simulink model "FOCFullSpeedControl"  (R2020b)
settings: Solver=ode4  StartTime=0.0  StopTime=4  FixedStep=1e-6  RelTol=1e-3
values from neighbouring files (symbols this model uses):
  E = 700    [FOCinit.m]
  f = 0.005    [FOCinit.m]
  J = 0.006    [FOCinit.m]
  Kie = 3 / (t5e * Ke)    (= 216000)    [FOCinit.m]
  Kif = 3 / (t5f * Kf)    (= 254.237288136)    [FOCinit.m]
  Kim = 3 / (t5m * Km)    (= 0.03)    [FOCinit.m]
  Kpe = taue * Kie    (= 2830.4)    [FOCinit.m]
  Kpf = tauf * Kif    (= 14.1242937853)    [FOCinit.m]
  Kpm = taum * Kim    (= 0.036)    [FOCinit.m]
  Lr = 0.075    [FOCinit.m]
  Ls = 0.280    (= 0.28)    [FOCinit.m]
  Msr = 0.118    [FOCinit.m]
  P = 2    [FOCinit.m]
  Rr = 1.35    [FOCinit.m]
  Rs = 7.2    [FOCinit.m]
  Ts = 1/fs    (= 0.0001)    [FOCinit.m]
libraries: mcbcontrolslib x6, slpidlib x4, simulink x1
settings Model: SimulationMode=accelerator  Creator=guillaume  LastModifiedBy=SF54888
settings DataIOCC: ReturnWorkspaceOutputs=off
settings DebuggingCC: ArithmeticOperatorsInVariantConditions=warning
settings SFSimCC: SimUseLocalCustomCode=off  CustomCodeUndefinedFunction=UseInterfaceOnly
settings RTWCC: RTWUseLocalCustomCode=off
settings CodeAppCC: StateflowObjectComments=on

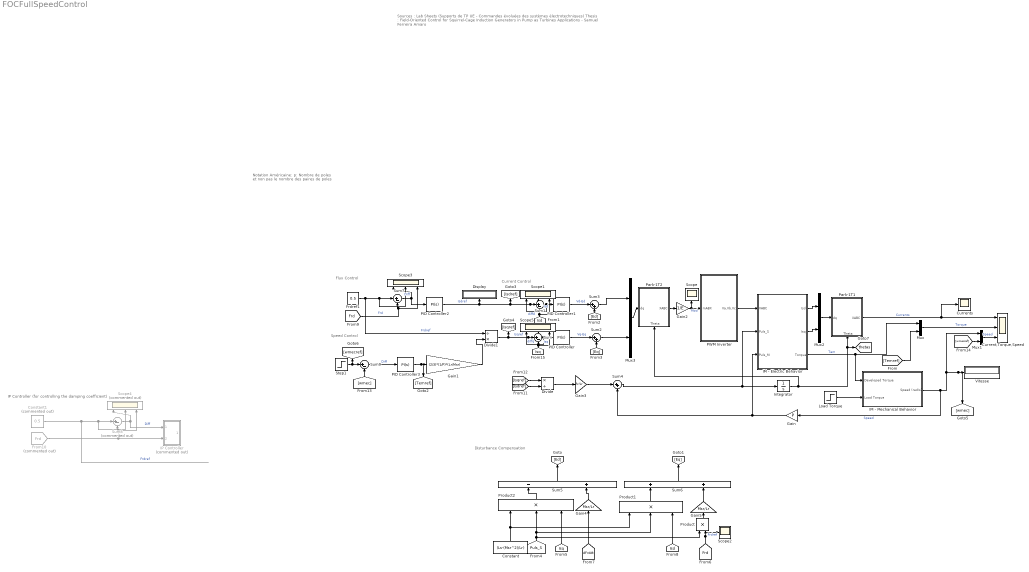
== system FOCFullSpeedControl ==
  note: Sources :
      | Lab Sheets (Supports de TP UE - Commandes évoluées des systèmes électrotechniques)
      | Thesis : Field-Oriented Control for Squirrel-Cage Induction Generators in Pump as Turbines Applications - Samuel Ferreira Amaro
  note: Notation Américaine:
      | p: Nombre de poles et
      | non pas le nombre des paires de poles
  note: Current Control
  note: Disturbance Compensation
  note: Speed Control
  note: IP Controller (for controlling the damping coefficient)
  note: Flux Control
  Constant : Constant  Value=(Ls-(Msr^2)/Lr)
  Constant1 : Constant  Commented=on  Value=0.5
  Current,Torque,Speed : Scope  NumInputPorts=3
  Currents : Scope
  Display : Display
  Divide : Product  Inputs=*/
  Divide1 : Product  Inputs=/*
  Frdref1 : Constant  Value=0.5
  From10 : From  Commented=on  GotoTag=Frd  TagVisibility=global
  Gain : Gain  Gain=P
  Gain1 : Gain  Gain=(2/3)*(1/P)*(Lr/Msr)
  Gain2 : Gain  Gain=1/E
  Gain3 : Gain  Gain=Rr/Lr
  Gain4 : Gain  Gain=Msr/Lr
  Gain5 : Gain  Gain=Msr/Lr
  IM - Electric Behavior : Subsystem
  IM - Mechanical Behavior : Subsystem
  IP Controller : Subsystem  Commented=on
  Integrator : Integrator
  Load Torque : Step  Time=2  After=0.5  SampleTime=0
  Mux{,1..3} (4 alike) : Mux  Inputs=2
  PID Controller : slpidlib/PID Controller  Controller=PI  Form=Parallel  TimeDomain=Continuous-time  UseExternalTs=off  SampleTime=-1  IntegratorMethod=Forward Euler  FilterMethod=Forward Euler  ControllerParametersSource=internal  P=Kpe  I=Kie  D=0  UseFilter=on  N=100  TunerSelectOption=Transfer Function Based (PID Tuner App)  InitialConditionSource=internal  InitialConditionForIntegrator=0  InitialConditionForFilter=0  DifferentiatorICPrevScaledInput=0  ExternalReset=none  TrackingMode=off  Kt=1  LimitOutput=off  SatLimitsSource=internal  UpperSaturationLimit=inf  LowerSaturationLimit=-inf  LinearizeAsGain=on  AntiWindupMode=none  Kb=1  POutMin=[]  POutMax=[]  IOutMin=[]  IOutMax=[]  DOutMin=[]  DOutMax=[]  NOutMin=[]  NOutMax=[]  SumOutMin=[]  SumOutMax=[]  SaturationOutMin=[]  SaturationOutMax=[]  PParamMin=[]  PParamMax=[]  IParamMin=[]  IParamMax=[]  DParamMin=[]  DParamMax=[]  NParamMin=[]  NParamMax=[]  KbParamMin=[]  KbParamMax=[]  KtParamMin=[]  KtParamMax=[]  KbOutMin=[]  KbOutMax=[]  KtOutMin=[]  KtOutMax=[]  IntegratorOutMin=[]  IntegratorOutMax=[]  FilterOutMin=[]  FilterOutMax=[]  SumI1OutMin=[]  SumI1OutMax=[]  SumI2OutMin=[]  SumI2OutMax=[]  SumI3OutMin=[]  SumI3OutMax=[]  SumI4OutMin=[]  SumI4OutMax=[]  SumDOutMin=[]  SumDOutMax=[]  DifferentiatorOutMin=[]  DifferentiatorOutMax=[]  FilterDiffOutCoefMin=[]  FilterDiffOutCoefMax=[]  ReciprocalOutMin=[]  ReciprocalOutMax=[]  SumDenOutMin=[]  SumDenOutMax=[]  SumNumOutMin=[]  SumNumOutMax=[]  DivideOutMin=[]  DivideOutMax=[]  UdiffTsProdOutMin=[]  UdiffTsProdOutMax=[]  NTsProdOutMin=[]  NTsProdOutMax=[]  UintegralTsProdOutMin=[]  UintegralTsProdOutMax=[]  UngainTsProdOutMin=[]  UngainTsProdOutMax=[]  IntegratorContinuousStateAttributes=''  IntegratorStateMustResolveToSignalObject=off  IntegratorRTWStateStorageClass=Auto  FilterContinuousStateAttributes=''  FilterStateMustResolveToSignalObject=off  FilterRTWStateStorageClass=Auto  ParallelPVariant=InternalParameters  IdealPVariant=Disabled  IVariant=InternalParameters  DVariant=Disabled  IntegratorVariant=Continuous  SatVariant=Disabled  AWVariant=Passthrough  PCopyVariant=Disabled  TRVariant=Disabled  FdbkBlocksVariant=Forward  IdealPFdbkVariant=Disabled  SatFdbkVariant=Disabled  DerivativeFilterVariant=Disabled  NVariant=Disabled  NCopyVariant=Disabled_SignalSpec  FilterICVariant=Disabled  IntegratorICVariant=InternalICs  ExternalResetVariant=Disabled  TRSumVariant=Passthrough  SumFdbkVariant=Disabled  SumVariant=Sum_PI  TsampFilterVariant=InternalTs  TsampNgainVariant=Passthrough  TsampIntegralVariant=Passthrough  ExternalSaturationOutDataTypeStr=Inherit: Same as second input
  PID Controller1 : slpidlib/PID Controller  Controller=PI  Form=Parallel  TimeDomain=Continuous-time  UseExternalTs=off  SampleTime=-1  IntegratorMethod=Forward Euler  FilterMethod=Forward Euler  ControllerParametersSource=internal  P=Kpe  I=Kie  D=0  UseFilter=on  N=100  TunerSelectOption=Transfer Function Based (PID Tuner App)  InitialConditionSource=internal  InitialConditionForIntegrator=0  InitialConditionForFilter=0  DifferentiatorICPrevScaledInput=0  ExternalReset=none  TrackingMode=off  Kt=1  LimitOutput=off  SatLimitsSource=internal  UpperSaturationLimit=inf  LowerSaturationLimit=-inf  LinearizeAsGain=on  AntiWindupMode=none  Kb=1  POutMin=[]  POutMax=[]  IOutMin=[]  IOutMax=[]  DOutMin=[]  DOutMax=[]  NOutMin=[]  NOutMax=[]  SumOutMin=[]  SumOutMax=[]  SaturationOutMin=[]  SaturationOutMax=[]  PParamMin=[]  PParamMax=[]  IParamMin=[]  IParamMax=[]  DParamMin=[]  DParamMax=[]  NParamMin=[]  NParamMax=[]  KbParamMin=[]  KbParamMax=[]  KtParamMin=[]  KtParamMax=[]  KbOutMin=[]  KbOutMax=[]  KtOutMin=[]  KtOutMax=[]  IntegratorOutMin=[]  IntegratorOutMax=[]  FilterOutMin=[]  FilterOutMax=[]  SumI1OutMin=[]  SumI1OutMax=[]  SumI2OutMin=[]  SumI2OutMax=[]  SumI3OutMin=[]  SumI3OutMax=[]  SumI4OutMin=[]  SumI4OutMax=[]  SumDOutMin=[]  SumDOutMax=[]  DifferentiatorOutMin=[]  DifferentiatorOutMax=[]  FilterDiffOutCoefMin=[]  FilterDiffOutCoefMax=[]  ReciprocalOutMin=[]  ReciprocalOutMax=[]  SumDenOutMin=[]  SumDenOutMax=[]  SumNumOutMin=[]  SumNumOutMax=[]  DivideOutMin=[]  DivideOutMax=[]  UdiffTsProdOutMin=[]  UdiffTsProdOutMax=[]  NTsProdOutMin=[]  NTsProdOutMax=[]  UintegralTsProdOutMin=[]  UintegralTsProdOutMax=[]  UngainTsProdOutMin=[]  UngainTsProdOutMax=[]  IntegratorContinuousStateAttributes=''  IntegratorStateMustResolveToSignalObject=off  IntegratorRTWStateStorageClass=Auto  FilterContinuousStateAttributes=''  FilterStateMustResolveToSignalObject=off  FilterRTWStateStorageClass=Auto  ParallelPVariant=InternalParameters  IdealPVariant=Disabled  IVariant=InternalParameters  DVariant=Disabled  IntegratorVariant=Continuous  SatVariant=Disabled  AWVariant=Passthrough  PCopyVariant=Disabled  TRVariant=Disabled  FdbkBlocksVariant=Forward  IdealPFdbkVariant=Disabled  SatFdbkVariant=Disabled  DerivativeFilterVariant=Disabled  NVariant=Disabled  NCopyVariant=Disabled_SignalSpec  FilterICVariant=Disabled  IntegratorICVariant=InternalICs  ExternalResetVariant=Disabled  TRSumVariant=Passthrough  SumFdbkVariant=Disabled  SumVariant=Sum_PI  TsampFilterVariant=InternalTs  TsampNgainVariant=Passthrough  TsampIntegralVariant=Passthrough  ExternalSaturationOutDataTypeStr=Inherit: Same as second input
  PID Controller2 : slpidlib/PID Controller  Controller=PI  Form=Parallel  TimeDomain=Continuous-time  UseExternalTs=off  SampleTime=-1  IntegratorMethod=Forward Euler  FilterMethod=Forward Euler  ControllerParametersSource=internal  P=Kpf  I=Kif  D=0  UseFilter=on  N=100  TunerSelectOption=Transfer Function Based (PID Tuner App)  InitialConditionSource=internal  InitialConditionForIntegrator=0  InitialConditionForFilter=0  DifferentiatorICPrevScaledInput=0  ExternalReset=none  TrackingMode=off  Kt=1  LimitOutput=off  SatLimitsSource=internal  UpperSaturationLimit=inf  LowerSaturationLimit=-inf  LinearizeAsGain=on  AntiWindupMode=none  Kb=1  POutMin=[]  POutMax=[]  IOutMin=[]  IOutMax=[]  DOutMin=[]  DOutMax=[]  NOutMin=[]  NOutMax=[]  SumOutMin=[]  SumOutMax=[]  SaturationOutMin=[]  SaturationOutMax=[]  PParamMin=[]  PParamMax=[]  IParamMin=[]  IParamMax=[]  DParamMin=[]  DParamMax=[]  NParamMin=[]  NParamMax=[]  KbParamMin=[]  KbParamMax=[]  KtParamMin=[]  KtParamMax=[]  KbOutMin=[]  KbOutMax=[]  KtOutMin=[]  KtOutMax=[]  IntegratorOutMin=[]  IntegratorOutMax=[]  FilterOutMin=[]  FilterOutMax=[]  SumI1OutMin=[]  SumI1OutMax=[]  SumI2OutMin=[]  SumI2OutMax=[]  SumI3OutMin=[]  SumI3OutMax=[]  SumI4OutMin=[]  SumI4OutMax=[]  SumDOutMin=[]  SumDOutMax=[]  DifferentiatorOutMin=[]  DifferentiatorOutMax=[]  FilterDiffOutCoefMin=[]  FilterDiffOutCoefMax=[]  ReciprocalOutMin=[]  ReciprocalOutMax=[]  SumDenOutMin=[]  SumDenOutMax=[]  SumNumOutMin=[]  SumNumOutMax=[]  DivideOutMin=[]  DivideOutMax=[]  UdiffTsProdOutMin=[]  UdiffTsProdOutMax=[]  NTsProdOutMin=[]  NTsProdOutMax=[]  UintegralTsProdOutMin=[]  UintegralTsProdOutMax=[]  UngainTsProdOutMin=[]  UngainTsProdOutMax=[]  IntegratorContinuousStateAttributes=''  IntegratorStateMustResolveToSignalObject=off  IntegratorRTWStateStorageClass=Auto  FilterContinuousStateAttributes=''  FilterStateMustResolveToSignalObject=off  FilterRTWStateStorageClass=Auto  ParallelPVariant=InternalParameters  IdealPVariant=Disabled  IVariant=InternalParameters  DVariant=Disabled  IntegratorVariant=Continuous  SatVariant=Disabled  AWVariant=Passthrough  PCopyVariant=Disabled  TRVariant=Disabled  FdbkBlocksVariant=Forward  IdealPFdbkVariant=Disabled  SatFdbkVariant=Disabled  DerivativeFilterVariant=Disabled  NVariant=Disabled  NCopyVariant=Disabled_SignalSpec  FilterICVariant=Disabled  IntegratorICVariant=InternalICs  ExternalResetVariant=Disabled  TRSumVariant=Passthrough  SumFdbkVariant=Disabled  SumVariant=Sum_PI  TsampFilterVariant=InternalTs  TsampNgainVariant=Passthrough  TsampIntegralVariant=Passthrough  ExternalSaturationOutDataTypeStr=Inherit: Same as second input
  PID Controller3 : slpidlib/PID Controller  Controller=PI  Form=Parallel  TimeDomain=Continuous-time  UseExternalTs=off  SampleTime=-1  IntegratorMethod=Forward Euler  FilterMethod=Forward Euler  ControllerParametersSource=internal  P=Kpm  I=Kim  D=0  UseFilter=on  N=100  TunerSelectOption=Transfer Function Based (PID Tuner App)  InitialConditionSource=internal  InitialConditionForIntegrator=0  InitialConditionForFilter=0  DifferentiatorICPrevScaledInput=0  ExternalReset=none  TrackingMode=off  Kt=1  LimitOutput=off  SatLimitsSource=internal  UpperSaturationLimit=inf  LowerSaturationLimit=-inf  LinearizeAsGain=on  AntiWindupMode=none  Kb=1  POutMin=[]  POutMax=[]  IOutMin=[]  IOutMax=[]  DOutMin=[]  DOutMax=[]  NOutMin=[]  NOutMax=[]  SumOutMin=[]  SumOutMax=[]  SaturationOutMin=[]  SaturationOutMax=[]  PParamMin=[]  PParamMax=[]  IParamMin=[]  IParamMax=[]  DParamMin=[]  DParamMax=[]  NParamMin=[]  NParamMax=[]  KbParamMin=[]  KbParamMax=[]  KtParamMin=[]  KtParamMax=[]  KbOutMin=[]  KbOutMax=[]  KtOutMin=[]  KtOutMax=[]  IntegratorOutMin=[]  IntegratorOutMax=[]  FilterOutMin=[]  FilterOutMax=[]  SumI1OutMin=[]  SumI1OutMax=[]  SumI2OutMin=[]  SumI2OutMax=[]  SumI3OutMin=[]  SumI3OutMax=[]  SumI4OutMin=[]  SumI4OutMax=[]  SumDOutMin=[]  SumDOutMax=[]  DifferentiatorOutMin=[]  DifferentiatorOutMax=[]  FilterDiffOutCoefMin=[]  FilterDiffOutCoefMax=[]  ReciprocalOutMin=[]  ReciprocalOutMax=[]  SumDenOutMin=[]  SumDenOutMax=[]  SumNumOutMin=[]  SumNumOutMax=[]  DivideOutMin=[]  DivideOutMax=[]  UdiffTsProdOutMin=[]  UdiffTsProdOutMax=[]  NTsProdOutMin=[]  NTsProdOutMax=[]  UintegralTsProdOutMin=[]  UintegralTsProdOutMax=[]  UngainTsProdOutMin=[]  UngainTsProdOutMax=[]  IntegratorContinuousStateAttributes=''  IntegratorStateMustResolveToSignalObject=off  IntegratorRTWStateStorageClass=Auto  FilterContinuousStateAttributes=''  FilterStateMustResolveToSignalObject=off  FilterRTWStateStorageClass=Auto  ParallelPVariant=InternalParameters  IdealPVariant=Disabled  IVariant=InternalParameters  DVariant=Disabled  IntegratorVariant=Continuous  SatVariant=Disabled  AWVariant=Passthrough  PCopyVariant=Disabled  TRVariant=Disabled  FdbkBlocksVariant=Forward  IdealPFdbkVariant=Disabled  SatFdbkVariant=Disabled  DerivativeFilterVariant=Disabled  NVariant=Disabled  NCopyVariant=Disabled_SignalSpec  FilterICVariant=Disabled  IntegratorICVariant=InternalICs  ExternalResetVariant=Disabled  TRSumVariant=Passthrough  SumFdbkVariant=Disabled  SumVariant=Sum_PI  TsampFilterVariant=InternalTs  TsampNgainVariant=Passthrough  TsampIntegralVariant=Passthrough  ExternalSaturationOutDataTypeStr=Inherit: Same as second input
  PWM Inverter : Subsystem
  Park-1T1 : Subsystem
      settings: PortSchema="{\"entries\":[{\"content\":{\"sides\":[{\"content\":{\"connectorIds\":[\"In1\"]},\"type\":\"ConnectorPlacement.EquallySpacedRectSide\",\"uuid\":\"c9ca9a07-e30b-41ed-8e45-9927ea626236\"},{\"content\":{\"connectorIds\":[\"Out1\"],\"side\":\"RIGHT\"},\"type\":\"ConnectorPlacement.EquallySpacedRectSide\",\"uuid\":\"8fc3e4f4-8f75-483a-a7a4-7af5e29f18e2\"},{\"content\":{\"connectorIds\":[],\"side\":\"TOP\"},\"type\":\"ConnectorPlacement.EquallySpacedRectSide\",\"uuid\":\"905320dc-39b9-4906-81e8-9c5e0c8b831b\"},{\"content\":{\"connectorIds\":[\"In2\"],\"side\":\"BOTTOM\"},\"type\":\"ConnectorPlacement.EquallySpacedRectSide\",\"uuid\":\"722fe21e-e1d8-480f-a57c-3b393e27675b\"},{\"content\":{\"connectorIds\":[],\"side\":\"HIDDEN\"},\"type\":\"ConnectorPlacement.EquallySpacedRectSide\",\"uuid\":\"f2f3dc36-ba2b-4cec-8f31-13e96319fff4\"}]},\"type\":\"ConnectorPlacement.EquallySpacedConnector\",\"uuid\":\"64f5051a-e69f-4636-88bd-017ed8687e6b\"}],\"packageUris\":[\"http://schema.mathworks.com/mf0/Connector/R2020b\"],\"version\":\"1.0\"}"
  Park-1T2 : Subsystem
      settings: PortSchema="{\"entries\":[{\"content\":{\"sides\":[{\"content\":{\"connectorIds\":[\"In1\"]},\"type\":\"ConnectorPlacement.EquallySpacedRectSide\",\"uuid\":\"c9ca9a07-e30b-41ed-8e45-9927ea626236\"},{\"content\":{\"connectorIds\":[\"Out1\"],\"side\":\"RIGHT\"},\"type\":\"ConnectorPlacement.EquallySpacedRectSide\",\"uuid\":\"8fc3e4f4-8f75-483a-a7a4-7af5e29f18e2\"},{\"content\":{\"connectorIds\":[],\"side\":\"TOP\"},\"type\":\"ConnectorPlacement.EquallySpacedRectSide\",\"uuid\":\"905320dc-39b9-4906-81e8-9c5e0c8b831b\"},{\"content\":{\"connectorIds\":[\"In2\"],\"side\":\"BOTTOM\"},\"type\":\"ConnectorPlacement.EquallySpacedRectSide\",\"uuid\":\"722fe21e-e1d8-480f-a57c-3b393e27675b\"},{\"content\":{\"connectorIds\":[],\"side\":\"HIDDEN\"},\"type\":\"ConnectorPlacement.EquallySpacedRectSide\",\"uuid\":\"f2f3dc36-ba2b-4cec-8f31-13e96319fff4\"}]},\"type\":\"ConnectorPlacement.EquallySpacedConnector\",\"uuid\":\"64f5051a-e69f-4636-88bd-017ed8687e6b\"}],\"packageUris\":[\"http://schema.mathworks.com/mf0/Connector/R2020b\"],\"version\":\"1.0\"}"
  Product : Product
  Product1 : Product  Inputs=3
  Product2 : Product  Inputs=3
  Scope : Scope
  Scope1 : Scope  NumInputPorts=3
  Scope2 : Scope
  Scope3 : Scope  NumInputPorts=3
  Scope4 : Scope  Commented=on  NumInputPorts=3
  Scope5 : Scope  NumInputPorts=3
  Step1 : Step  After=150  SampleTime=0
  Sum{,1,7,9} (4 alike) : Sum  Inputs=|+-
  Sum2 : Sum  Inputs=|++
  Sum3 : Sum  Inputs=|++
  Sum4 : Sum  Inputs=|++
  Sum5 : Sum  Inputs=-+
  Sum6 : Sum
  Sum8 : Sum  Commented=on  Inputs=|+-
  Vitesse : Display
  tag scope: thetas=global
  wires:
  Load Torque/1 -> IM - Mechanical Behavior/2(Load Torque)
  Gain/1 -> Sum4/2, IM - Electric Behavior/3(Puls_M)
  IM - Electric Behavior/1(Isd) -> Mux2/1
  IM - Electric Behavior/2(Isq) -> Mux2/2
  Park-1T1/1(XABC) -> Currents/1, Current,Torque,Speed/1  "Currents"
  IM - Electric Behavior/3(Torque) -> Mux/1, IM - Mechanical Behavior/1(Developed Torque)  "Tem"
  IM - Mechanical Behavior/1(Speed (rad/s)) -> Mux1/1, [wmec], Vitesse/1, Gain/1  "Speed"
  Mux2/1 -> Park-1T1/1(dq)
  Gain1/1 -> Divide1/2
  Divide1/1 -> [Isqref], Scope5/2, Sum/1  "Isqref"
  Sum1/1 -> PID Controller1/1, Scope1/1  "diffd"
  PID Controller/1 -> Sum2/1  "Vq-Eq"
  PID Controller1/1 -> Sum3/1  "Vd-Ed"
  Sum3/1 -> Mux3/1
  Sum2/1 -> Mux3/2
  Divide/1 -> Gain3/1
  Gain3/1 -> Sum4/1
  Sum4/1 -> IM - Electric Behavior/2(Puls_S), Integrator/1
  Integrator/1 -> Park-1T1/2(Theta), [thetas], Park-1T2/2(Theta)
  [Ed] -> Sum3/2
  [Eq] -> Sum2/2
  Sum5/1 -> [Ed]
  [Isd] -> Scope1/3, Sum1/2  "Isd"
  Sum/1 -> Scope5/1, PID Controller/1  "diffq"
  [Isq] -> Scope5/3, Sum/2  "Isq"
  [Temref] -> Mux/2
  Mux/1 -> Current,Torque,Speed/2  "Torque"
  [dFrddt] -> Gain4/1
  Gain4/1 -> Sum5/2
  Constant/1 -> Product2/1, Product1/1
  [Puls_S] -> Product1/2, Product2/2, Product/1
  [Isq] -> Product2/3
  Product2/1 -> Sum5/1
  [Isd] -> Product1/3
  Product1/1 -> Sum6/1
  Gain5/1 -> Sum6/2
  Product/1 -> Gain5/1
  Sum6/1 -> [Eq]
  PID Controller3/1 -> [Temref], Gain1/1
  [Frd] -> Scope2/1, Product/2  "Frdref"
  PID Controller2/1 -> [Isdref], Scope1/2, Sum1/1, Display/1  "Isdref"
  [Isdref] -> Divide/2
  [Isqref] -> Divide/1
  Sum9/1 -> PID Controller3/1  "Diff"
  [wmec] -> Sum9/2
  Step1/1 -> Sum9/1, [wmecref]
  Mux1/1 -> Current,Torque,Speed/3  "Speed"
  [wmecref] -> Mux1/2
  Mux3/1 -> Park-1T2/1(dq)
  Gain2/1 -> Scope/1, PWM Inverter/1(mABX)  "Mod"
  Park-1T2/1(XABC) -> Gain2/1
  PWM Inverter/1(Va,Vb,Vc) -> IM - Electric Behavior/1(VABC)
  Constant1/1 -> Scope4/2, Sum8/1  "Frdref"
  From10/1 -> IP Controller/2(meas), Scope4/3, Sum8/2
  Sum8/1 -> IP Controller/1(Diff), Scope4/1  "Diff"
  [Frd] -> Scope3/3, Sum7/2  "Frd"
  Frdref1/1 -> Divide1/1, Scope3/2, Sum7/1  "Frdref"
  Sum7/1 -> PID Controller2/1, Scope3/1  "Diff"

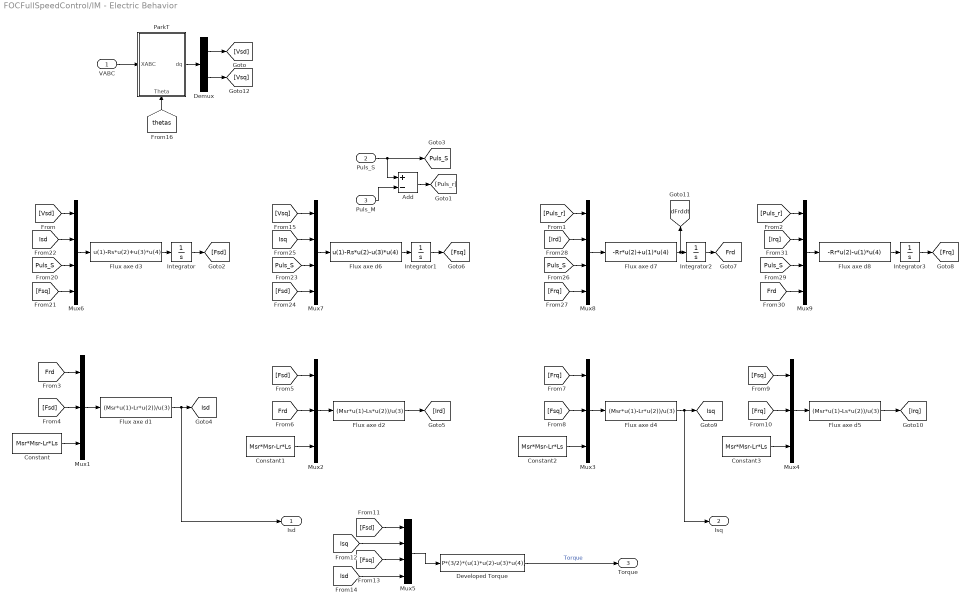
== system FOCFullSpeedControl/IM - Electric Behavior ==
  VABC : Inport
  Puls_S : Inport  Port=2
  Puls_M : Inport  Port=3
  Add : Sum  Inputs=+-
  Constant{,1..3} (4 alike) : Constant  Value=Msr*Msr-Lr*Ls
  Demux : Demux  Outputs=2
  Developed Torque : Fcn  Expr=P*(3/2)*(u(1)*u(2)-u(3)*u(4))
  Flux axe d1 : Fcn  Expr=(Msr*u(1)-Lr*u(2))/u(3)
  Flux axe d2 : Fcn  Expr=(Msr*u(1)-Ls*u(2))/u(3)
  Flux axe d3 : Fcn  Expr=u(1)-Rs*u(2)+u(3)*u(4)
  Flux axe d4 : Fcn  Expr=(Msr*u(1)-Lr*u(2))/u(3)
  Flux axe d5 : Fcn  Expr=(Msr*u(1)-Ls*u(2))/u(3)
  Flux axe d6 : Fcn  Expr=u(1)-Rs*u(2)-u(3)*u(4)
  Flux axe d7 : Fcn  Expr=-Rr*u(2)+u(1)*u(4)
  Flux axe d8 : Fcn  Expr=-Rr*u(2)-u(1)*u(4)
  Integrator{,1..3} (4 alike) : Integrator
  Mux{1..4} (4 alike) : Mux  Inputs=3
  Mux{5..9} (5 alike) : Mux
  ParkT : Subsystem
      settings: PortSchema="{\"entries\":[{\"content\":{\"sides\":[{\"content\":{\"connectorIds\":[\"In1\"]},\"type\":\"ConnectorPlacement.EquallySpacedRectSide\",\"uuid\":\"c9ca9a07-e30b-41ed-8e45-9927ea626236\"},{\"content\":{\"connectorIds\":[\"Out1\"],\"side\":\"RIGHT\"},\"type\":\"ConnectorPlacement.EquallySpacedRectSide\",\"uuid\":\"8fc3e4f4-8f75-483a-a7a4-7af5e29f18e2\"},{\"content\":{\"connectorIds\":[],\"side\":\"TOP\"},\"type\":\"ConnectorPlacement.EquallySpacedRectSide\",\"uuid\":\"905320dc-39b9-4906-81e8-9c5e0c8b831b\"},{\"content\":{\"connectorIds\":[\"In2\"],\"side\":\"BOTTOM\"},\"type\":\"ConnectorPlacement.EquallySpacedRectSide\",\"uuid\":\"413e78c1-b829-4cef-8159-d6b0dd019bd4\"},{\"content\":{\"connectorIds\":[],\"side\":\"HIDDEN\"},\"type\":\"ConnectorPlacement.EquallySpacedRectSide\",\"uuid\":\"f2f3dc36-ba2b-4cec-8f31-13e96319fff4\"}]},\"type\":\"ConnectorPlacement.EquallySpacedConnector\",\"uuid\":\"64f5051a-e69f-4636-88bd-017ed8687e6b\"}],\"packageUris\":[\"http://schema.mathworks.com/mf0/Connector/R2020b\"],\"version\":\"1.0\"}"
  Isd : Outport
  Isq : Outport  Port=2
  Torque : Outport  Port=3
  tag scope: Frd=global, Isd=global, Isq=global, Puls_S=global, dFrddt=global
  wires:
  Puls_S/1 -> Add/1, [Puls_S]
  Mux6/1 -> Flux axe d3/1
  [Vsd] -> Mux6/1
  [Isd] -> Mux6/2
  [Puls_S] -> Mux6/3
  [Fsq] -> Mux6/4
  Flux axe d3/1 -> Integrator/1
  Integrator/1 -> [Fsd]
  Mux7/1 -> Flux axe d6/1
  [Vsq] -> Mux7/1
  [Isq] -> Mux7/2
  [Puls_S] -> Mux7/3
  [Fsd] -> Mux7/4
  Flux axe d6/1 -> Integrator1/1
  Integrator1/1 -> [Fsq]
  Mux8/1 -> Flux axe d7/1
  [Ird] -> Mux8/2
  [Puls_S] -> Mux8/3
  [Frq] -> Mux8/4
  Flux axe d7/1 -> [dFrddt], Integrator2/1
  Integrator2/1 -> [Frd]
  Mux9/1 -> Flux axe d8/1
  [Puls_r] -> Mux8/1
  [Irq] -> Mux9/2
  [Puls_S] -> Mux9/3
  [Frd] -> Mux9/4
  Flux axe d8/1 -> Integrator3/1
  Integrator3/1 -> [Frq]
  [Puls_r] -> Mux9/1
  [Frd] -> Mux1/1
  [Fsd] -> Mux1/2
  Mux1/1 -> Flux axe d1/1
  Constant/1 -> Mux1/3
  Flux axe d1/1 -> Isd/1, [Isd]
  [Fsd] -> Mux2/1
  [Frd] -> Mux2/2
  Mux2/1 -> Flux axe d2/1
  Constant1/1 -> Mux2/3
  Flux axe d2/1 -> [Ird]
  [Frq] -> Mux3/1
  [Fsq] -> Mux3/2
  Mux3/1 -> Flux axe d4/1
  Constant2/1 -> Mux3/3
  Flux axe d4/1 -> Isq/1, [Isq]
  [Fsq] -> Mux4/1
  [Frq] -> Mux4/2
  Mux4/1 -> Flux axe d5/1
  Constant3/1 -> Mux4/3
  Flux axe d5/1 -> [Irq]
  Mux5/1 -> Developed Torque/1
  Developed Torque/1 -> Torque/1  "Torque"
  [Isd] -> Mux5/4
  [Fsd] -> Mux5/1
  [Isq] -> Mux5/2
  [Fsq] -> Mux5/3
  Puls_M/1 -> Add/2
  Add/1 -> [Puls_r]
  VABC/1 -> ParkT/1(XABC)
  Demux/2 -> [Vsq]
  Demux/1 -> [Vsd]
  ParkT/1(dq) -> Demux/1
  [thetas] -> ParkT/2(Theta)

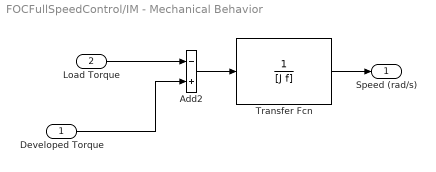
== system FOCFullSpeedControl/IM - Mechanical Behavior ==
  Developed Torque : Inport
  Load Torque : Inport  Port=2
  Add2 : Sum  Inputs=-+
  Transfer Fcn : TransferFcn  Denominator=[J f]
  Speed (rad/s) : Outport
  wires:
  Developed Torque/1 -> Add2/2
  Load Torque/1 -> Add2/1
  Add2/1 -> Transfer Fcn/1
  Transfer Fcn/1 -> Speed (rad/s)/1

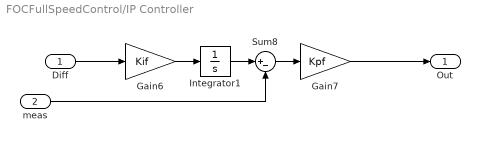
== system FOCFullSpeedControl/IP Controller ==
  Diff : Inport
  meas : Inport  Port=2
  Gain6 : Gain  Gain=Kif
  Gain7 : Gain  Gain=Kpf
  Integrator1 : Integrator  InitialCondition=0.5/Msr
  Sum8 : Sum  Inputs=|+-
  Out : Outport
  wires:
  Sum8/1 -> Gain7/1
  Integrator1/1 -> Sum8/1
  Gain6/1 -> Integrator1/1
  Diff/1 -> Gain6/1
  meas/1 -> Sum8/2
  Gain7/1 -> Out/1

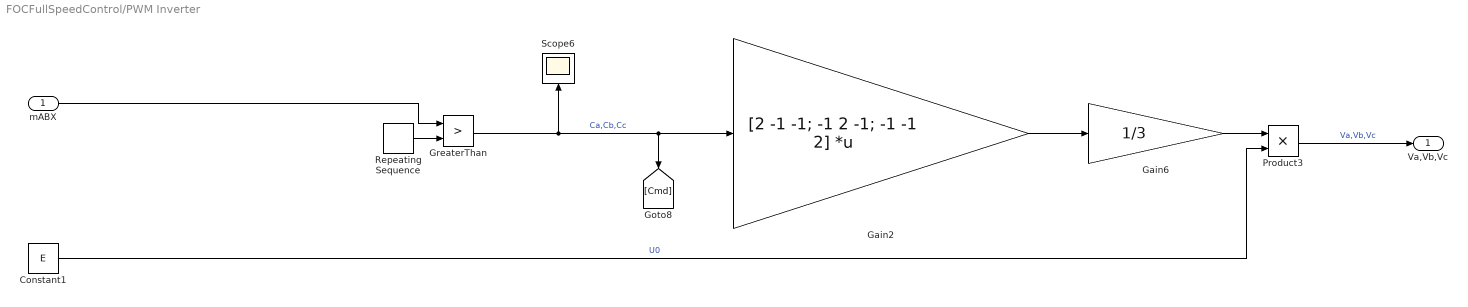
== system FOCFullSpeedControl/PWM Inverter ==
  mABX : Inport
  Constant1 : Constant  Value=E
  Gain2 : Gain  Gain=[2 -1 -1; -1 2 -1; -1 -1 2]  Multiplication=Matrix(K*u)
  Gain6 : Gain  Gain=1/3
  GreaterThan : RelationalOperator  Operator=>  OutDataTypeStr=boolean  RndMeth=Simplest
  Product3 : Product
  Repeating Sequence : simulink/Sources/Repeating Sequence  rep_seq_t=[0 Ts]  rep_seq_y=[-1 1]
  Scope6 : Scope
  Va,Vb,Vc : Outport
  wires:
  Gain2/1 -> Gain6/1
  Product3/1 -> Va,Vb,Vc/1  "Va,Vb,Vc"
  mABX/1 -> GreaterThan/1
  GreaterThan/1 -> [Cmd], Gain2/1, Scope6/1  "Ca,Cb,Cc"
  Repeating Sequence/1 -> GreaterThan/2
  Constant1/1 -> Product3/2  "U0"
  Gain6/1 -> Product3/1

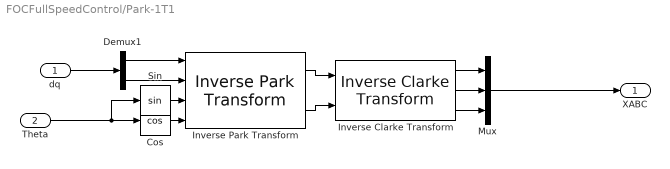
== system FOCFullSpeedControl/Park-1T1 ==
  dq : Inport
  Theta : Inport  Port=2
  Cos : Trigonometry  Operator=cos
  Demux1 : Demux  Outputs=2
  Inverse Clarke Transform : mcbcontrolslib/Inverse Clarke Transform
      settings: SourceProductBaseCode=MT
  Inverse Park Transform : mcbcontrolslib/Inverse Park Transform  AxisAlignment=D-axis
  Mux : Mux  Inputs=3
  Sin : Trigonometry
  XABC : Outport
  wires:
  Inverse Park Transform/2 -> Inverse Clarke Transform/2
  Demux1/2 -> Inverse Park Transform/2
  dq/1 -> Demux1/1
  Inverse Clarke Transform/1 -> Mux/1
  Inverse Park Transform/1 -> Inverse Clarke Transform/1
  Demux1/1 -> Inverse Park Transform/1
  Theta/1 -> Sin/1, Cos/1
  Inverse Clarke Transform/2 -> Mux/2
  Cos/1 -> Inverse Park Transform/4
  Sin/1 -> Inverse Park Transform/3
  Inverse Clarke Transform/3 -> Mux/3
  Mux/1 -> XABC/1

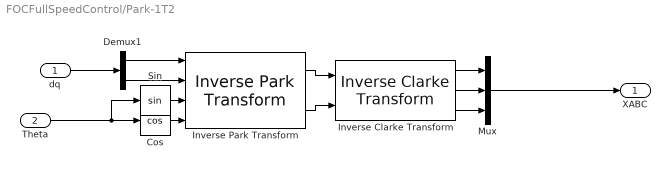
== system FOCFullSpeedControl/Park-1T2 ==
  dq : Inport
  Theta : Inport  Port=2
  Cos : Trigonometry  Operator=cos
  Demux1 : Demux  Outputs=2
  Inverse Clarke Transform : mcbcontrolslib/Inverse Clarke Transform
      settings: SourceProductBaseCode=MT
  Inverse Park Transform : mcbcontrolslib/Inverse Park Transform  AxisAlignment=D-axis
  Mux : Mux  Inputs=3
  Sin : Trigonometry
  XABC : Outport
  wires:
  Inverse Park Transform/2 -> Inverse Clarke Transform/2
  Demux1/2 -> Inverse Park Transform/2
  dq/1 -> Demux1/1
  Inverse Clarke Transform/1 -> Mux/1
  Inverse Park Transform/1 -> Inverse Clarke Transform/1
  Demux1/1 -> Inverse Park Transform/1
  Theta/1 -> Sin/1, Cos/1
  Inverse Clarke Transform/2 -> Mux/2
  Cos/1 -> Inverse Park Transform/4
  Sin/1 -> Inverse Park Transform/3
  Inverse Clarke Transform/3 -> Mux/3
  Mux/1 -> XABC/1

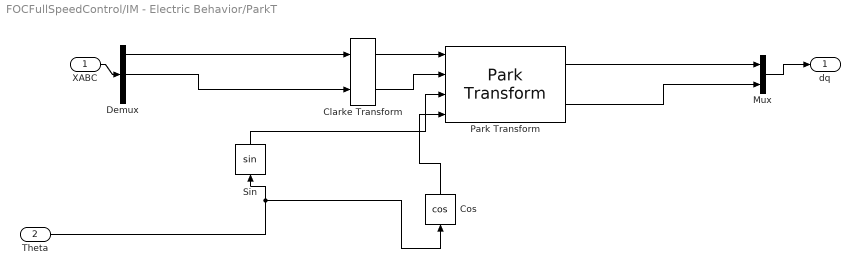
== system FOCFullSpeedControl/IM - Electric Behavior/ParkT ==
  XABC : Inport
  Theta : Inport  Port=2
  Clarke Transform : mcbcontrolslib/Clarke Transform  VariantControl=Variant2
  Cos : Trigonometry  Operator=cos
  Demux : Demux  Outputs=3
  Mux : Mux  Inputs=2
  Park Transform : mcbcontrolslib/Park Transform  AxisAlignment=D-axis
      settings: SourceProductBaseCode=MT
  Sin : Trigonometry
  dq : Outport
  wires:
  Park Transform/2 -> Mux/2
  Demux/2 -> Clarke Transform/2
  Sin/1 -> Park Transform/3
  Theta/1 -> Sin/1, Cos/1
  Clarke Transform/2 -> Park Transform/2
  Clarke Transform/1 -> Park Transform/1
  Cos/1 -> Park Transform/4
  Park Transform/1 -> Mux/1
  Demux/1 -> Clarke Transform/1
  XABC/1 -> Demux/1
  Mux/1 -> dq/1
